simulink model "waterTank"  (Simulink 9.1)
settings: Solver=ode45  StartTime=0.0  StopTime=560.0  FixedStep=1  RelTol=1e-3  EnableMultiTasking=on
settings Model: SuppressorTable=22 serialization::archive 11 0 6 0 0 0 1 0  Creator=yangg  LastModifiedBy=wangjian
settings DataIOCC: LimitDataPoints=on
settings DebuggingCC: UnderspecifiedInitializationDetection=Simplified  MergeDetectMultiDrivingBlocksExec=error  SolverPrmCheckMsg=warning
settings GRTTargetCC: GeneratePreprocessorConditionals=Disable all  CombineOutputUpdateFcns=on  GRTInterface=off
settings ConfigComp: CovSFcnEnable=off

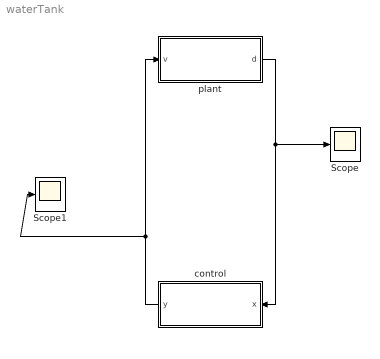
== system waterTank ==
  Scope : Scope
  Scope1 : Scope
  control : Subsystem
  plant : Subsystem
  wires:
  plant/1(d) -> Scope/1, control/1(x)
  control/1(y) -> Scope1/1, plant/1(v)

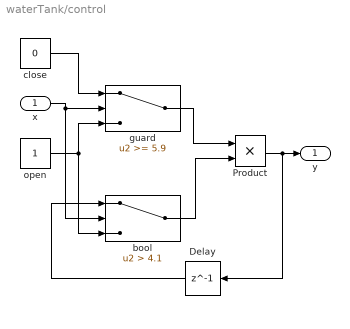
== system waterTank/control ==
  x : Inport  SampleTime=1
  Delay : Delay  DelayLength=1  InitialCondition=0
  Product : Product  SampleTime=1
  bool : Switch  Criteria=u2 > Threshold  Threshold=4.1  SampleTime=1
  close : Constant  Value=0  SampleTime=1
  guard : Switch  Threshold=5.9  SampleTime=1
  open : Constant  SampleTime=1
  y : Outport  SampleTime=1
  wires:
  close/1 -> guard/1
  x/1 -> bool/2, guard/2
  open/1 -> bool/3, guard/3
  guard/1 -> Product/1
  bool/1 -> Product/2
  Product/1 -> Delay/1, y/1
  Delay/1 -> bool/1

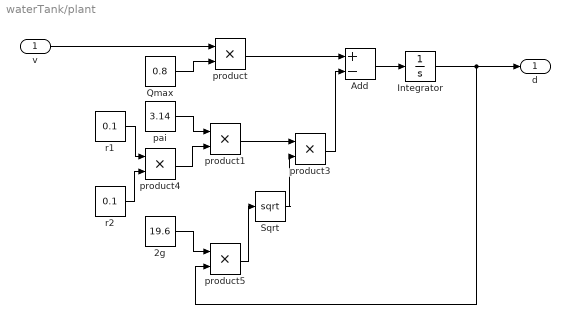
== system waterTank/plant ==
  v : Inport
  2g : Constant  Value=19.6
  Add : Sum  Inputs=+-  SampleTime=0
  Integrator : Integrator  InitialCondition=5
  Qmax : Constant  Value=0.8
  Sqrt : Sqrt  SampleTime=0  SaturateOnIntegerOverflow=on
  pai : Constant  Value=3.14
  product{,1,3..5} (5 alike) : Product  Inputs=**  SampleTime=0
  r1 : Constant  Value=0.1
  r2 : Constant  Value=0.1
  d : Outport
  wires:
  Qmax/1 -> product/2
  pai/1 -> product1/1
  product4/1 -> product1/2
  r1/1 -> product4/1
  r2/1 -> product4/2
  2g/1 -> product5/1
  product1/1 -> product3/1
  product/1 -> Add/1
  product3/1 -> Add/2
  Add/1 -> Integrator/1
  Integrator/1 -> d/1, product5/2
  product5/1 -> Sqrt/1
  Sqrt/1 -> product3/2
  v/1 -> product/1
